simulink model "simuQ3"  (R2016b)
settings: Solver=VariableStepAuto  StartTime=0.0  StopTime=10.0  RelTol=1e-3
libraries: simulink x1, aerolibatmos2 x1, aerolibconvert2 x1
settings Model: Creator=AP19030  LastModifiedBy=AP19030

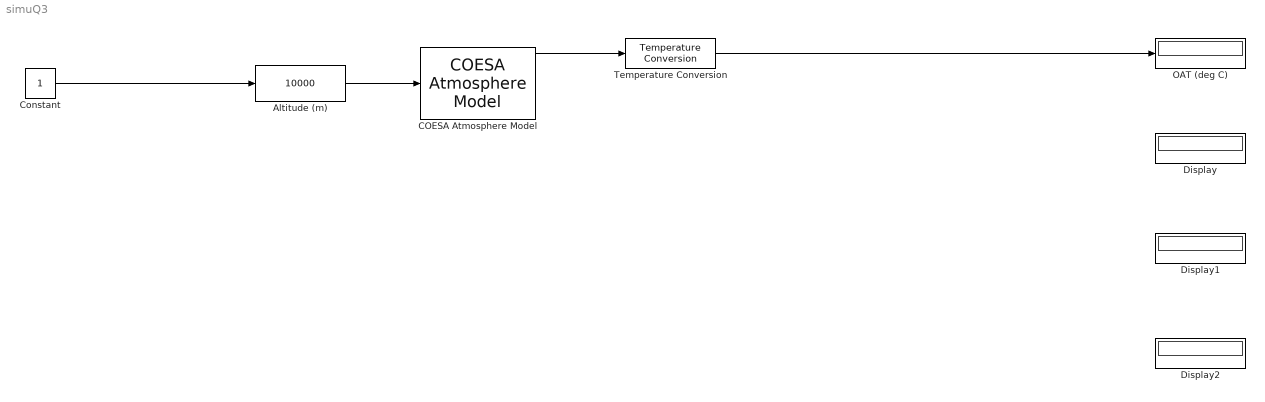
== system simuQ3 ==
  Altitude (m) : simulink/Math Operations/Slider Gain  low=0  gain=10000  high=10000
  COESA Atmosphere Model : aerolibatmos2/COESA Atmosphere Model  units=Metric (MKS)  spec=1976 COESA-extended U.S. Standard Atmosphere  model=Profile  profile_var=High temperature  profile_percent=1%  profile_alt=5 km (16404 ft)  envelope_var=High temperature  envelope_percent=1%  action=Warning
  Constant : Constant
  Display : Display
  Display1 : Display
  Display2 : Display
  OAT (deg C) : Display
      settings: Format=decimal (Stored Integer)  Decimation=50
  Temperature Conversion : aerolibconvert2/Temperature Conversion  IU=R  OU=K
  wires:
  Altitude (m)/1 -> COESA Atmosphere Model/1
  Constant/1 -> Altitude (m)/1
  COESA Atmosphere Model/1 -> Temperature Conversion/1
  Temperature Conversion/1 -> OAT (deg C)/1
